simulink model "Question10Hw1_AkankshaMurali"  (R2023b)
settings: Solver=VariableStepAuto  StartTime=0.0  StopTime=10.0  RelTol=1e-3
settings Model: Creator=shash  LastModifiedBy=akank

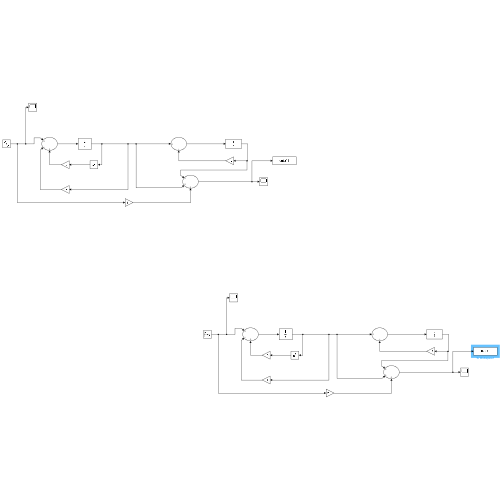
[thumbnail: Simulink's stored preview of the top-level diagram]
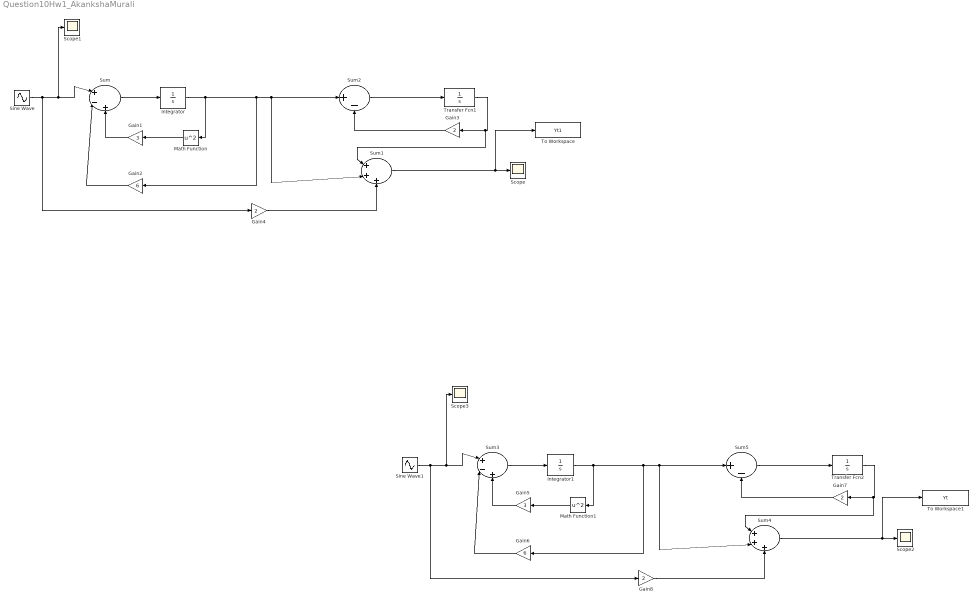
== system Question10Hw1_AkankshaMurali ==
  Gain1 : Gain  Gain=3
  Gain2 : Gain  Gain=6
  Gain{3..4,7..8} (4 alike) : Gain  Gain=2
  Gain5 : Gain  Gain=3
  Gain6 : Gain  Gain=6
  Integrator : Integrator
  Integrator1 : Integrator
  Math Function : Math  Operator=square
  Math Function1 : Math  Operator=square
  Scope{,1..3} (4 alike) : Scope
  Sine Wave : Sin  SampleTime=0
  Sine Wave1 : Sin  Amplitude=3  SampleTime=0
  Sum : Sum  Inputs=|+-+
  Sum1 : Sum  Inputs=|+++
  Sum2 : Sum  Inputs=|+-
  Sum3 : Sum  Inputs=|+-+
  Sum4 : Sum  Inputs=|+++
  Sum5 : Sum  Inputs=|+-
  To Workspace : ToWorkspace  VariableName=Yt1  SaveFormat=Timeseries  SampleTime=-1
  To Workspace1 : ToWorkspace  VariableName=Yt  SaveFormat=Timeseries  SampleTime=-1
  Transfer Fcn1 : TransferFcn  Denominator=[1 0]
  Transfer Fcn2 : TransferFcn  Denominator=[1 0]
  wires:
  Sum/1 -> Integrator/1
  Math Function/1 -> Gain1/1
  Integrator/1 -> Sum2/1, Sum1/2, Gain2/1, Math Function/1
  Sine Wave/1 -> Gain4/1, Scope1/1, Sum/1
  Gain1/1 -> Sum/3
  Gain2/1 -> Sum/2
  Gain4/1 -> Sum1/3
  Sum2/1 -> Transfer Fcn1/1
  Transfer Fcn1/1 -> Sum1/1, Gain3/1
  Gain3/1 -> Sum2/2
  Sum1/1 -> To Workspace/1, Scope/1
  Transfer Fcn2/1 -> Sum4/1, Gain7/1
  Sum5/1 -> Transfer Fcn2/1
  Gain8/1 -> Sum4/3
  Sum3/1 -> Integrator1/1
  Integrator1/1 -> Sum5/1, Sum4/2, Gain6/1, Math Function1/1
  Sum4/1 -> To Workspace1/1, Scope2/1
  Gain7/1 -> Sum5/2
  Gain5/1 -> Sum3/3
  Math Function1/1 -> Gain5/1
  Gain6/1 -> Sum3/2
  Sine Wave1/1 -> Gain8/1, Scope3/1, Sum3/1
